simulink model "linear_pendulum"  (R2018a)
settings: Solver=VariableStepAuto  StartTime=0.0  StopTime=10.0  RelTol=1e-3
values from neighbouring files (symbols this model uses):
  c = 0.25    [linear_pendulum_plot.m]    (also in pendulum.m)
  g = 9.81    [linear_pendulum_plot.m]    (also in pendulum.m)
  l = 2    [linear_pendulum_plot.m]    (also in pendulum.m)
  m = 1    [linear_pendulum_plot.m]    (also in pendulum.m)
settings Model: Creator=ee128-aaz  LastModifiedBy=ee128-aaz

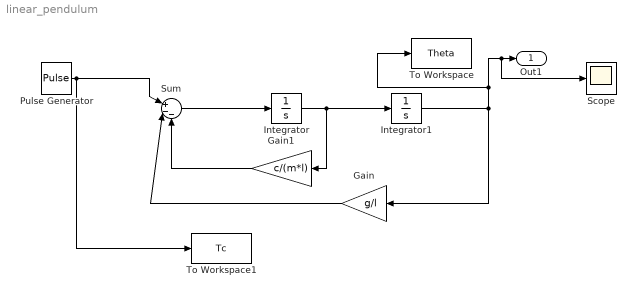
== system linear_pendulum ==
  Gain : Gain  Gain=g/l
  Gain1 : Gain  Gain=c/(m*l)
  Integrator : Integrator
  Integrator1 : Integrator
  Pulse Generator : DiscretePulseGenerator  PulseType=Time based  Amplitude=10  Period=100  PulseWidth=0.2
  Scope : Scope
  Sum : Sum  Inputs=|+--
  To Workspace : ToWorkspace  VariableName=Theta  SaveFormat=Timeseries  SampleTime=-1
  To Workspace1 : ToWorkspace  VariableName=Tc  SaveFormat=Timeseries  SampleTime=-1
  Out1 : Outport
  wires:
  Sum/1 -> Integrator/1
  Pulse Generator/1 -> To Workspace1/1, Sum/1
  Gain1/1 -> Sum/3
  Integrator/1 -> Gain1/1, Integrator1/1
  Integrator1/1 -> Gain/1, Scope/1, Out1/1, To Workspace/1
  Gain/1 -> Sum/2
